simulink model "boostObserver_old"  (R2020a)
settings: Solver=VariableStepAuto  StartTime=0.0  StopTime=3.2  FixedStep=0.0005  MaxStep=9e-06  RelTol=1e-03  EnableMultiTasking=on
InitFcn:
  | kp=0.01;
  | ki=0.01;
  | 
  | k=2;
  | em=100000000;
  | GE=1/em;
  | GU=k*ki/GE;
  | GCE=k*kp/GU;
model workspace (MAT data in the model file):
  time = 0.8
values from neighbouring files (symbols this model uses):
  A1 = obj.boostConverter.A1    [BoostController.m]    (also in BoostConverter.m = [-obj.R/obj.L 0;0 -1/(obj.Ro*obj.C)]; BuckBoostConverter.m = [-obj.R/obj.L 0;0 -1/(obj.Ro*obj.C)]; obsmc.m = Asigma{1,1}; workspace_atual.mat = [-16.4  0; 0  -3.50877192982])
  A2 = obj.boostConverter.A2    [BoostController.m]    (also in BoostConverter.m = [-obj.R/obj.L -1/obj.L;1/obj.C -1/(obj.Ro*obj.C)]; BuckBoostConverter.m = [-obj.R/obj.L 1/obj.L;-1/obj.C -1/(obj.Ro*obj.C)]; obsmc.m = Asigma{1,2}; workspace_atual.mat = [-16.4  -200; 350.877192982  -3.50877192982])
  AlarmDeadTime = 0.50    (= 0.5)    [BoostFaultSimulation.m]    (also in workspace_atual.mat; workspace_certo.mat)
  B1 = obj.boostConverter.B1    [BoostController.m]    (also in BoostConverter.m = [1/obj.L;0]; BuckBoostConverter.m = [1/obj.L;0]; obsmc.m = Bsigma{1,1}; workspace_atual.mat = [200 0])
  boost_parameters = [obj.Ro,obj.R,obj.L,obj.C,obj.u]'    [BoostConverter.m]    (also in BuckBoostConverter.m; boostResults2Latex.m = boost.parameters(); workspace_atual.mat = [100 0.082 0.005 0.00285 190]; workspace_certo.mat = [100 0.082 0.005 0.00285 190])
  C = 1e-3    (= 0.001)    [boostResults2Latex.m]
  CiL = [0 1]    [workspace_atual.mat]    (also in workspace_certo.mat)
  Cmatrix = [1  0; 0  1]    [workspace_atual.mat]    (also in workspace_certo.mat)
  CVc = [1 0]    [workspace_atual.mat]    (also in workspace_certo.mat)
  D1 = [1  0; 0  1]    [workspace_atual.mat]    (also in workspace_certo.mat)
  FaultClass = 0    [BoostFaultSimulation.m]    (also in workspace_atual.mat = 1; workspace_certo.mat = 1)
  iLFaultSwitch = 0    [BoostFaultSimulation.m]    (also in workspace_atual.mat; workspace_certo.mat)
  iLFaultTime = 1.70    (= 1.7)    [BoostFaultSimulation.m]    (also in workspace_atual.mat; workspace_certo.mat)
  iLGainFaultFactor = 15    [BoostFaultSimulation.m]    (also in workspace_atual.mat; workspace_certo.mat)
  iLNoiseFaultSwitch = 0    [BoostFaultSimulation.m]    (also in workspace_atual.mat; workspace_certo.mat)
  iLNoiseTime = 1.70    (= 1.7)    [BoostFaultSimulation.m]    (also in workspace_atual.mat; workspace_certo.mat)
  Jth = 2000    [workspace_atual.mat]    (also in workspace_certo.mat)
  L = 1e-3    (= 0.001)    [boostResults2Latex.m]    (also in obsmc.m = sdpvar(3,1,'full'))
  LoadAddResistor = obj.LoadAddFactor*obj.Ro    [BoostFaultSimulation.m]    (also in workspace_atual.mat = 30; workspace_certo.mat = 30)
  LoadAddSignalSwitch = 1    [BoostFaultSimulation.m]    (also in workspace_atual.mat; workspace_certo.mat)
  LoadAddSwitch = 0    [BoostFaultSimulation.m]    (also in workspace_atual.mat; workspace_certo.mat)
  LoadAddTime = 0.90    (= 0.9)    [BoostFaultSimulation.m]    (also in workspace_atual.mat; workspace_certo.mat)
  LoadRemoveResistor = obj.Ro*(1-obj.LoadRemoveFactor)/(obj.LoadRemoveFactor)    [BoostFaultSimulation.m]    (also in workspace_atual.mat = 233.333333333; workspace_certo.mat = 233.333333333)
  LoadRemoveSignalSwitch = 1    [BoostFaultSimulation.m]    (also in workspace_atual.mat; workspace_certo.mat)
  LoadRemoveSwitch = 0    [BoostFaultSimulation.m]    (also in workspace_atual.mat; workspace_certo.mat)
  LoadRemoveTime = 0.90    (= 0.9)    [BoostFaultSimulation.m]    (also in workspace_atual.mat; workspace_certo.mat)
  LobsiL = [1737913.15707 66180.0912281]    [workspace_atual.mat]    (also in workspace_certo.mat)
  LobsVc = [61200 1]    [workspace_atual.mat]    (also in workspace_certo.mat)
  ObsEp = 70    [workspace_atual.mat]    (also in workspace_certo.mat)
  R = 0.1    [boostResults2Latex.m]    (also in workspace_atual.mat = 0.082; workspace_certo.mat = 0.082)
  ReconfigDelay = 0    [BoostFaultSimulation.m]    (also in workspace_atual.mat = 0.2; workspace_certo.mat = 0.2)
  ReconfigSwitch = 0    [BoostFaultSimulation.m]    (also in workspace_atual.mat; workspace_certo.mat)
  ReconfigTime = 1.707    [BoostFaultSimulation.m]    (also in workspace_atual.mat; workspace_certo.mat)
  rho = 5    [workspace_atual.mat]    (also in workspace_certo.mat)
  RMSfrequency = 47.61    [BoostFaultSimulation.m]    (also in workspace_atual.mat; workspace_certo.mat)
  Ro = 100    [BoostFaultSimulation.m]    (also in boostResults2Latex.m = 10; workspace_atual.mat; workspace_certo.mat)
  Smep = 80    [workspace_atual.mat]    (also in workspace_certo.mat)
  SourceAddSignalSwitch = 1    [BoostFaultSimulation.m]    (also in workspace_atual.mat; workspace_certo.mat)
  SourceAddSwitch = 0    [BoostFaultSimulation.m]    (also in workspace_atual.mat; workspace_certo.mat)
  SourceAddTime = 0.90    (= 0.9)    [BoostFaultSimulation.m]    (also in workspace_atual.mat; workspace_certo.mat)
  SourceAddVoltage = obj.SourceAddFactor*obj.u    [BoostFaultSimulation.m]    (also in workspace_atual.mat = 19; workspace_certo.mat = 19)
  SourceRemoveSignalSwitch = 1    [BoostFaultSimulation.m]    (also in workspace_atual.mat; workspace_certo.mat)
  SourceRemoveSwitch = 0    [BoostFaultSimulation.m]    (also in workspace_atual.mat; workspace_certo.mat)
  SourceRemoveTime = 0.90    (= 0.9)    [BoostFaultSimulation.m]    (also in workspace_atual.mat; workspace_certo.mat)
  SourceRemoveVoltage = obj.SourceRemoveFactor*obj.u    [BoostFaultSimulation.m]    (also in workspace_atual.mat = 19; workspace_certo.mat = 19)
  ueq = 0.5    [workspace_atual.mat]    (also in workspace_certo.mat)
  VcFaultSwitch = 0    [BoostFaultSimulation.m]    (also in workspace_atual.mat; workspace_certo.mat)
  VcFaultTime = 1.70    (= 1.7)    [BoostFaultSimulation.m]    (also in workspace_atual.mat; workspace_certo.mat)
  VcGainFaultFactor = 15    [BoostFaultSimulation.m]    (also in workspace_atual.mat; workspace_certo.mat)
  VcNoiseFaultSwitch = 0    [BoostFaultSimulation.m]    (also in workspace_atual.mat; workspace_certo.mat)
  VcNoiseTime = 1.70    (= 1.7)    [BoostFaultSimulation.m]    (also in workspace_atual.mat; workspace_certo.mat)
  ve = 380    [BoostFaultSimulation.m]    (also in boostResults2Latex.m = 100; workspace_atual.mat; workspace_certo.mat)
  x_e = [ie;ve]    [BoostConverter.m]    (also in BuckBoostConverter.m)
  xe = obj.boostConverter.equilibriumstate(ve)    [BoostController.m]    (also in workspace_atual.mat = [7.62509288104 380]; workspace_certo.mat = [7.62509288104 380])
undefined symbols (not defined in the file or in its folder): Atilde1, Atilde2, Ctilde1, Dtilde1, Dtilde2, F, G, MAXnet, MINnet
libraries: neural x74, powerlib x70, dspstat3 x16, simulink x9, powerlib_meascontrol x7, dspmtrx3 x7, dspmathops x3
(part 3 of 7)

== system boostObserver_old/Subsystem/D(f_s)/Subsystem2 ==
  input : Inport
  FaultStep : Inport  Port=2
  NoiseStep : Inport  Port=3
  FaultSwtich : Inport  Port=4
  NoiseFaultSwitch : Inport  Port=5
  FaultFactor : Inport  Port=6
  Constant11 : Constant  Value=0
  Constant9 : Constant  Value=0
  Product : Product
  Subsystem : Subsystem
  Switch10 : Switch  Criteria=u2 ~= 0
  Switch11 : Switch  Criteria=u2 ~= 0
  Switch13 : Switch  Criteria=u2 ~= 0
  Switch9 : Switch  Criteria=u2 ~= 0  ZeroCross=off
  iLFault Switch : MultiPortSwitch  DataPortOrder=Zero-based contiguous  DataPortForDefault=Additional data port  zeroidx=on
  output : Outport
  wires:
  input/1 -> Product/1, Switch11/3, iLFault Switch/2, Switch10/3, iLFault Switch/5
  Constant9/1 -> Switch10/1
  Switch13/1 -> Switch9/2
  Switch9/1 -> output/1
  Switch11/1 -> iLFault Switch/4
  Constant11/1 -> Switch13/3
  iLFault Switch/1 -> Switch9/3, Subsystem/1(input)
  Switch10/1 -> iLFault Switch/3
  FaultStep/1 -> Switch11/2, Switch10/2
  NoiseStep/1 -> Switch13/1
  FaultSwtich/1 -> iLFault Switch/1
  NoiseFaultSwitch/1 -> Switch13/2
  FaultFactor/1 -> Product/2
  Product/1 -> Switch11/1
  Subsystem/1(noiseOutput) -> Switch9/1

== system boostObserver_old/Subsystem/ErrorGenerator/If Action Subsystem ==
  e_y : Inport
  Action Port : ActionPort  ActionPortLabel=if(u1 ~= 0)
  Matrix Multiply : Product  Multiplication=Matrix(*)
  Matrix Multiply1 : Product
  Matrizes A1 : Constant  Value=rho
  Matrizes A2 : Constant  Value=F
  Normalization : dspmathops/Normalization  NormType=2-norm  Bias=1e-10  NormOver=Each column  Dimension=1  roundingMode=Floor  overflowMode=off  accumDataTypeStr=Inherit: Same as product output  accumLastDataTypeStr=Inherit: Same as product output  outputDataTypeStr=Inherit: Same as product output  outputMin=[]  outputMax=[]  outputLastDataTypeStr=Inherit: Same as product output
  v : Outport
  wires:
  Matrix Multiply/1 -> Normalization/1
  Matrizes A2/1 -> Matrix Multiply/1
  Normalization/1 -> Matrix Multiply1/2
  e_y/1 -> Matrix Multiply/2
  Matrizes A1/1 -> Matrix Multiply1/1
  Matrix Multiply1/1 -> v/1

== system boostObserver_old/Subsystem/ErrorGenerator/If Action Subsystem1 ==
  e_y : Inport
  Action Port : ActionPort  ActionPortLabel=else
  v : Outport
  wires:
  e_y/1 -> v/1

== system boostObserver_old/Subsystem/Fault Identification Neural Netowrk/Pattern Recognition Neural Network1 ==
  Input : Inport  PortDimensions=3
      mask Display: e = 0.06;c1 = [120 230 180]/255;c2 = ([120 230 180]+0)/(256+128);c3 = ([120 230 180]+128)/(256+128);patch([0 1 1 0],[0 0 1 1],c1);patch([0 1 1 1-e 1-e 0+e],[0 0 1 1-e 0+e 0+e],c2);patch([0 0 1 1-e 0+e 0+e],[0 1 1 1-e 1-e 0+e],c3);plot([0 1 1 0 0],[0 0 1 1 0]);
  Layer 1 : Subsystem
      mask Display: e = 0.06;c1 = [120 150 230]/255;c2 = ([120 150 230]+0)/383;c3 = ([120 150 230]+128)/383;patch([0 1 1 0],[0 0 1 1],c1);patch([0 1 1 1-e 1-e 0+e],[0 0 1 1-e 0+e 0+e],c2);patch([0 0 1 1-e 0+e 0+e],[0 1 1 1-e 1-e 0+e],c3);plot([0 1 1 0 0],[0 0 1 1 0]);
  Layer 2 : Subsystem
      mask Display: e = 0.06;c1 = [120 150 230]/255;c2 = ([120 150 230]+0)/383;c3 = ([120 150 230]+128)/383;patch([0 1 1 0],[0 0 1 1],c1);patch([0 1 1 1-e 1-e 0+e],[0 0 1 1-e 0+e 0+e],c2);patch([0 0 1 1-e 0+e 0+e],[0 1 1 1-e 1-e 0+e],c3);plot([0 1 1 0 0],[0 0 1 1 0]);
  Process Input 1 : Subsystem
      mask Display: e = 0.06;c1 = [120 150 230]/255;c2 = ([120 150 230]+0)/383;c3 = ([120 150 230]+128)/383;patch([0 1 1 0],[0 0 1 1],c1);patch([0 1 1 1-e 1-e 0+e],[0 0 1 1-e 0+e 0+e],c2);patch([0 0 1 1-e 0+e 0+e],[0 1 1 1-e 1-e 0+e],c3);plot([0 1 1 0 0],[0 0 1 1 0]);
  Process Output 1 : Subsystem
      mask Display: e = 0.06;c1 = [120 150 230]/255;c2 = ([120 150 230]+0)/383;c3 = ([120 150 230]+128)/383;patch([0 1 1 0],[0 0 1 1],c1);patch([0 1 1 1-e 1-e 0+e],[0 0 1 1-e 0+e 0+e],c2);patch([0 0 1 1-e 0+e 0+e],[0 1 1 1-e 1-e 0+e],c3);plot([0 1 1 0 0],[0 0 1 1 0]);
  Output : Outport  InitialOutput=[0;0;0;0;0]
      mask Display: e = 0.06;c1 = [120 230 180]/255;c2 = ([120 230 180]+0)/(256+128);c3 = ([120 230 180]+128)/(256+128);patch([0 1 1 0],[0 0 1 1],c1);patch([0 1 1 1-e 1-e 0+e],[0 0 1 1-e 0+e 0+e],c2);patch([0 0 1 1-e 0+e 0+e],[0 1 1 1-e 1-e 0+e],c3);plot([0 1 1 0 0],[0 0 1 1 0]);
  wires:
  Input/1 -> Process Input 1/1(x)
  Process Output 1/1(y) -> Output/1
  Process Input 1/1(p) -> Layer 1/1("p{1}")
  Layer 1/1("a{1}") -> [feedback1]
  [feedback1] -> Layer 2/1("a{1} ")
  Layer 2/1("a{2}") -> Process Output 1/1(a)

== system boostObserver_old/Subsystem/Fault Identification Neural Netowrk/Subsystem ==
  input : Inport
  min : Inport  Port=2
  max : Inport  Port=3
  Constant2 : Constant  Value=2
  Constant3 : Constant
  Divide : Product  Inputs=*/
  Product : Product
  Sum : Sum  Inputs=|+-
  Sum1 : Sum  Inputs=|+-
  Sum2 : Sum  Inputs=|+-
  Out1 : Outport
  wires:
  Divide/1 -> Product/2
  max/1 -> Sum2/1
  Constant3/1 -> Sum1/2
  Product/1 -> Sum1/1
  input/1 -> Sum/1
  Sum/1 -> Divide/1
  Sum2/1 -> Divide/2
  Constant2/1 -> Product/1
  Sum1/1 -> Out1/1
  min/1 -> Sum/2, Sum2/2

== system boostObserver_old/Subsystem/Fault Identification Neural Netowrk/Subsystem1 ==
  input : Inport
  min : Inport  Port=2
  max : Inport  Port=3
  Constant2 : Constant  Value=2
  Constant3 : Constant
  Divide : Product  Inputs=*/
  Product : Product
  Sum : Sum  Inputs=|+-
  Sum1 : Sum  Inputs=|+-
  Sum2 : Sum  Inputs=|+-
  Out1 : Outport
  wires:
  Divide/1 -> Product/2
  max/1 -> Sum2/1
  Constant3/1 -> Sum1/2
  Product/1 -> Sum1/1
  input/1 -> Sum/1
  Sum/1 -> Divide/1
  Sum2/1 -> Divide/2
  Constant2/1 -> Product/1
  Sum1/1 -> Out1/1
  min/1 -> Sum/2, Sum2/2

== system boostObserver_old/Subsystem/Fault Identification Neural Netowrk/Subsystem2 ==
  input : Inport
  min : Inport  Port=2
  max : Inport  Port=3
  Constant2 : Constant  Value=2
  Constant3 : Constant
  Divide : Product  Inputs=*/
  Product : Product
  Sum : Sum  Inputs=|+-
  Sum1 : Sum  Inputs=|+-
  Sum2 : Sum  Inputs=|+-
  Out1 : Outport
  wires:
  Divide/1 -> Product/2
  max/1 -> Sum2/1
  Constant3/1 -> Sum1/2
  Product/1 -> Sum1/1
  input/1 -> Sum/1
  Sum/1 -> Divide/1
  Sum2/1 -> Divide/2
  Constant2/1 -> Product/1
  Sum1/1 -> Out1/1
  min/1 -> Sum/2, Sum2/2

== system boostObserver_old/Subsystem/Sliding Mode Observer 5/ObserverDynamics ==
  ey : Inport
  v : Inport  Port=2
  sigma : Inport  Port=3
  Gain : Gain  Gain=Atilde1  Multiplication=Matrix(K*u)
  Gain1 : Gain  Gain=G  Multiplication=Matrix(K*u)
  Gain3 : Gain  Gain=Dtilde1  Multiplication=Matrix(K*u)
  Gain5 : Gain  Gain=Atilde2  Multiplication=Matrix(K*u)
  Gain7 : Gain  Gain=Dtilde2  Multiplication=Matrix(K*u)
  Integral : Subsystem
  Sum : Sum  Inputs=|+++
  Sum1 : Sum  Inputs=|+++
  Switch1 : Switch  Criteria=u2 > Threshold
  e_tilde_hat : Outport
  wires:
  sigma/1 -> Switch1/2
  Switch1/1 -> Integral/1(e_hat_dot)  "v"
  Integral/1(e_hat) -> Gain/1, e_tilde_hat/1, Gain5/1
  ey/1 -> Gain1/1
  v/1 -> Gain7/1, Gain3/1
  Sum1/1 -> Switch1/3
  Sum/1 -> Switch1/1
  Gain7/1 -> Sum1/2
  Gain5/1 -> Sum1/3
  Gain3/1 -> Sum/1
  Gain1/1 -> Sum1/1, Sum/2
  Gain/1 -> Sum/3

== system boostObserver_old/Subsystem/Subsystem/SlidingSurface ==
  S : Inport
  ep : Inport  Port=2
  Abs : Abs  ZeroCross=off
  GreaterThan : RelationalOperator  Operator=>  OutDataTypeStr=boolean  RndMeth=Simplest
  If : If  IfExpression=u1 ~= 0
  If Action Subsystem : Subsystem  TreatAsAtomicUnit=on
  If Action Subsystem2 : Subsystem  TreatAsAtomicUnit=on
  Merge1 : Merge
  d : Outport
  wires:
  If Action Subsystem2/1(d) -> Merge1/2
  [S] -> If Action Subsystem/1(S), If Action Subsystem2/1(S)
  If/2 -> If Action Subsystem2/Action
  If/1 -> If Action Subsystem/Action
  [ep] -> If Action Subsystem2/2(ep)
  S/1 -> [S], Abs/1
  If Action Subsystem/1(d) -> Merge1/1
  Abs/1 -> GreaterThan/1
  GreaterThan/1 -> If/1
  Merge1/1 -> d/1
  ep/1 -> [ep], GreaterThan/2

== system boostObserver_old/Subsystem/Subsystem1/SlidingSurface ==
  S : Inport
  ep : Inport  Port=2
  Abs : Abs  ZeroCross=off
  GreaterThan : RelationalOperator  Operator=>  OutDataTypeStr=boolean  RndMeth=Simplest
  If : If  IfExpression=u1 ~= 0
  If Action Subsystem : Subsystem  TreatAsAtomicUnit=on
  If Action Subsystem2 : Subsystem  TreatAsAtomicUnit=on
  Merge1 : Merge
  d : Outport
  wires:
  If Action Subsystem2/1(d) -> Merge1/2
  [S] -> If Action Subsystem/1(S), If Action Subsystem2/1(S)
  If/2 -> If Action Subsystem2/Action
  If/1 -> If Action Subsystem/Action
  [ep] -> If Action Subsystem2/2(ep)
  S/1 -> [S], Abs/1
  If Action Subsystem/1(d) -> Merge1/1
  Abs/1 -> GreaterThan/1
  GreaterThan/1 -> If/1
  Merge1/1 -> d/1
  ep/1 -> [ep], GreaterThan/2

== system boostObserver_old/Subsystem/Subsystem9/Residual Generator2 ==
  e_y : Inport
  Matrix Square1 : dspmtrx3/Matrix Square  OutMin=[]  OutMax=[]
      settings: SourceProductBaseCode=DS
  Moving RMS : dspstat3/Moving RMS  Method=Sliding window  ForgettingFactorPort=off  SpecifyWindowLength=on  WindowLength=RMSfrequency/10  ForgettingFactor=0.9  SimulateUsing=Code generation
      settings: SourceProductBaseCode=DS
  Sqrt2 : Sqrt  SaturateOnIntegerOverflow=on
  RMS : Outport
  wires:
  Matrix Square1/1 -> Sqrt2/1
  e_y/1 -> Matrix Square1/1
  Sqrt2/1 -> Moving RMS/1
  Moving RMS/1 -> RMS/1

== system boostObserver_old/Subsystem/Vc OBserver/calc_x_hat ==
  sigma : Inport
  rsign : Inport  Port=2
  Lobs : Inport  Port=3
  Gain : Gain  Gain=A1  Multiplication=Matrix(K*u)
  Gain5 : Gain  Gain=A2  Multiplication=Matrix(K*u)
  Integral : Subsystem
  Matrix Multiply : Product  Multiplication=Matrix(*)
  MatrizesA8 : Constant  Value=B1*u
  Scope1 : Scope
  Sum : Sum  Inputs=|+++
  Sum1 : Sum  Inputs=|+++
  Switch1 : Switch  Criteria=u2 ~= 0
  x_hat : Outport
  wires:
  sigma/1 -> Switch1/2
  Switch1/1 -> Integral/1(x_hat_dot)  "v"
  Integral/1(x_hat) -> Scope1/1, x_hat/1, Gain/1, Gain5/1
  Sum1/1 -> Switch1/3
  Sum/1 -> Switch1/1
  Gain/1 -> Sum/3
  Gain5/1 -> Sum1/3
  Matrix Multiply/1 -> Sum/2, Sum1/2
  MatrizesA8/1 -> Sum1/1, Sum/1
  Lobs/1 -> Matrix Multiply/1
  rsign/1 -> Matrix Multiply/2

== system boostObserver_old/Subsystem/iL Observer/calc_x_hat ==
  sigma : Inport
  rsign : Inport  Port=2
  Lobs : Inport  Port=3
  Gain : Gain  Gain=A1  Multiplication=Matrix(K*u)
  Gain5 : Gain  Gain=A2  Multiplication=Matrix(K*u)
  Integral : Subsystem
  Matrix Multiply : Product  Multiplication=Matrix(*)
  MatrizesA8 : Constant  Value=B1*u
  Scope1 : Scope
  Sum : Sum  Inputs=|+++
  Sum1 : Sum  Inputs=|+++
  Switch1 : Switch  Criteria=u2 ~= 0
  x_hat : Outport
  wires:
  sigma/1 -> Switch1/2
  Switch1/1 -> Integral/1(x_hat_dot)  "v"
  Integral/1(x_hat) -> Scope1/1, x_hat/1, Gain/1, Gain5/1
  Sum1/1 -> Switch1/3
  Sum/1 -> Switch1/1
  Gain/1 -> Sum/3
  Gain5/1 -> Sum1/3
  Matrix Multiply/1 -> Sum/2, Sum1/2
  MatrizesA8/1 -> Sum1/1, Sum/1
  Lobs/1 -> Matrix Multiply/1
  rsign/1 -> Matrix Multiply/2

== system boostObserver_old/Subsystem3/Augmented Error Generator/z1 ==
  z_dot : Inport
  Constant1 : Constant  Value=[0;0]  VectorParams1D=off
  Gain2 : Gain  Gain=Cmatrix  Multiplication=Matrix(K*u) (u vector)
  Integrator6 : Integrator  InitialConditionSource=external
  z : Outport
  wires:
  Gain2/1 -> Integrator6/1
  Integrator6/1 -> z/1
  z_dot/1 -> Gain2/1
  Constant1/1 -> Integrator6/2

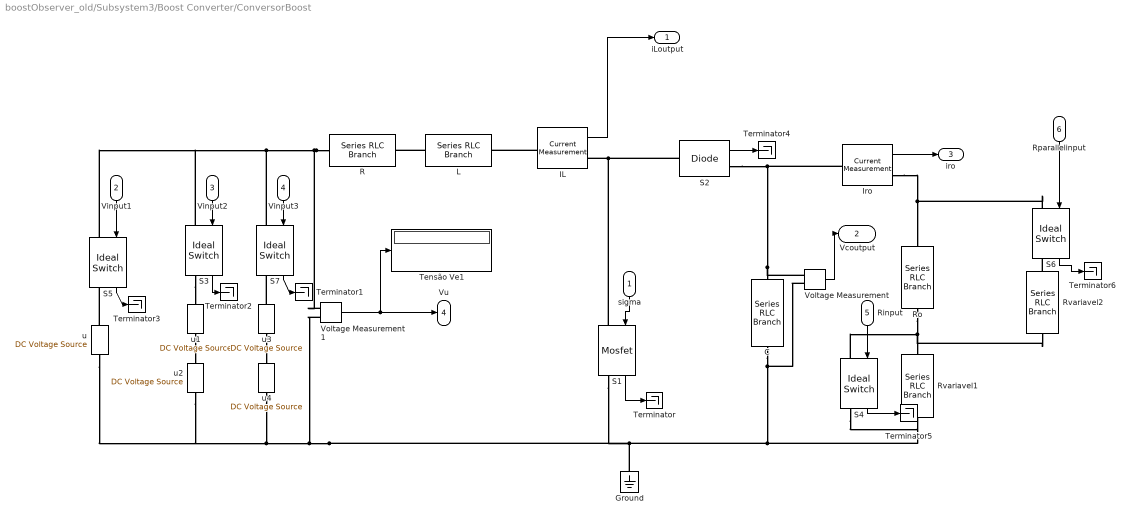
== system boostObserver_old/Subsystem3/Boost Converter/ConversorBoost ==
  sigma : Inport
  Vinput1 : Inport  Port=2
  Vinput2 : Inport  Port=3
  Vinput3 : Inport  Port=4
  Rinput : Inport  Port=5
  Rparallelinput : Inport  Port=6
  C : powerlib/Elements/Series RLC Branch  LConnTagsString=__new0  RConnTagsString=__new0  BranchType=C  Resistance=1  Inductance=1e-3  SetiL0=off  InitialCurrent=0  Capacitance=C  Setx0=on  InitialVoltage=0  Measurements=None
  Ground : powerlib/Elements/Ground  LConnTagsString=a
  IL : powerlib/Measurements/Current Measurement  PhasorSimulation=off  OutputType=Complex  PSBequivalent=0
  Iro : powerlib/Measurements/Current Measurement  PhasorSimulation=off  OutputType=Complex  PSBequivalent=0
  L : powerlib/Elements/Series RLC Branch  LConnTagsString=__new0  RConnTagsString=__new0  BranchType=L  Resistance=1  Inductance=L  SetiL0=on  InitialCurrent=0  Capacitance=1e-6  Setx0=off  InitialVoltage=0  Measurements=None
  R : powerlib/Elements/Series RLC Branch  LConnTagsString=__new0  RConnTagsString=__new0  BranchType=R  Resistance=R  Inductance=1e-3  SetiL0=off  InitialCurrent=0  Capacitance=1e-6  Setx0=off  InitialVoltage=0  Measurements=None
  Ro : powerlib/Elements/Series RLC Branch  LConnTagsString=__new0  RConnTagsString=__new0  BranchType=R  Resistance=Ro  Inductance=1e-3  SetiL0=off  InitialCurrent=0  Capacitance=1e-6  Setx0=off  InitialVoltage=0  Measurements=None
  Rvariavel1 : powerlib/Elements/Series RLC Branch  LConnTagsString=__new0  RConnTagsString=__new0  BranchType=R  Resistance=LoadAddResistor  Inductance=1e-3  SetiL0=off  InitialCurrent=0  Capacitance=1e-6  Setx0=off  InitialVoltage=0  Measurements=None
  Rvariavel2 : powerlib/Elements/Series RLC Branch  LConnTagsString=__new0  RConnTagsString=__new0  BranchType=R  Resistance=LoadRemoveResistor  Inductance=1e-3  SetiL0=off  InitialCurrent=0  Capacitance=1e-6  Setx0=off  InitialVoltage=0  Measurements=None
  S1 : powerlib/Power Electronics/Mosfet  Ron=0.0000001  Lon=0  Rd=0.000000001  Vfd=0  IC=0  Rs=1e5  Cs=inf  Measurements=on
  S2 : powerlib/Power Electronics/Diode  Ron=0.000001  Lon=0  Vf=0  IC=0  UseSnubber=off  Rs=0  Cs=0  Measurements=on
  S{3..7} (5 alike) : powerlib/Power Electronics/Ideal Switch  Ron=0.0000001  Lon=0  IC=0  Rs=1e8  Cs=inf  Measurements=on
  Tensão Ve1 : Display
  Terminator{,1..6} (7 alike) : Terminator
  Voltage Measurement : powerlib/Measurements/Voltage Measurement  PhasorSimulation=off  OutputType=Complex  PSBequivalent=0
  Voltage Measurement1 : powerlib/Measurements/Voltage Measurement  PhasorSimulation=off  OutputType=Complex  PSBequivalent=0
  u : powerlib/Electrical Sources/DC Voltage Source  Amplitude=u  Measurements=None
  u1 : powerlib/Electrical Sources/DC Voltage Source  Amplitude=SourceAddVoltage  Measurements=None
  u2 : powerlib/Electrical Sources/DC Voltage Source  Amplitude=u  Measurements=None
  u3 : powerlib/Electrical Sources/DC Voltage Source  Amplitude=SourceRemoveVoltage  Measurements=None
  u4 : powerlib/Electrical Sources/DC Voltage Source  Amplitude=u  Measurements=None
  iLoutput : Outport
  Vcoutput : Outport  Port=2
  iro : Outport  Port=3
  Vu : Outport  Port=4
  wires:
  Rinput/1 -> S4/1
  IL/1 -> iLoutput/1
  sigma/1 -> S1/1
  Voltage Measurement/1 -> Vcoutput/1
  Iro/1 -> iro/1
  Voltage Measurement1/1 -> Vu/1, Tensão Ve1/1
  Vinput1/1 -> S5/1
  Vinput2/1 -> S3/1
  Rparallelinput/1 -> S6/1
  Vinput3/1 -> S7/1
  S1/1 -> Terminator/1
  S7/1 -> Terminator1/1
  S3/1 -> Terminator2/1
  S5/1 -> Terminator3/1
  S2/1 -> Terminator4/1
  S4/1 -> Terminator5/1
  S6/1 -> Terminator6/1
  connections:
  Ro/RConn1 -- Rvariavel2/LConn1 -- Rvariavel1/RConn1 -- S4/LConn1
  IL/LConn1 -- L/RConn1
  C/RConn1 -- S4/RConn1 -- Rvariavel1/LConn1 -- S1/RConn1 -- u2/LConn1 -- u/LConn1 -- u4/LConn1 -- Voltage Measurement1/LConn2 -- Ground/LConn1 -- Voltage Measurement/LConn2
  S2/LConn1 -- S1/LConn1 -- IL/RConn1
  R/LConn1 -- S3/LConn1 -- S5/LConn1 -- S7/LConn1 -- Voltage Measurement1/LConn1
  Iro/RConn1 -- S6/LConn1 -- Ro/LConn1
  L/LConn1 -- R/RConn1
  S2/RConn1 -- Iro/LConn1 -- Voltage Measurement/LConn1 -- C/LConn1
  u/RConn1 -- S5/RConn1
  Rvariavel2/RConn1 -- S6/RConn1
  S3/RConn1 -- u1/RConn1
  u1/LConn1 -- u2/RConn1
  u3/LConn1 -- S7/RConn1
  u3/RConn1 -- u4/RConn1

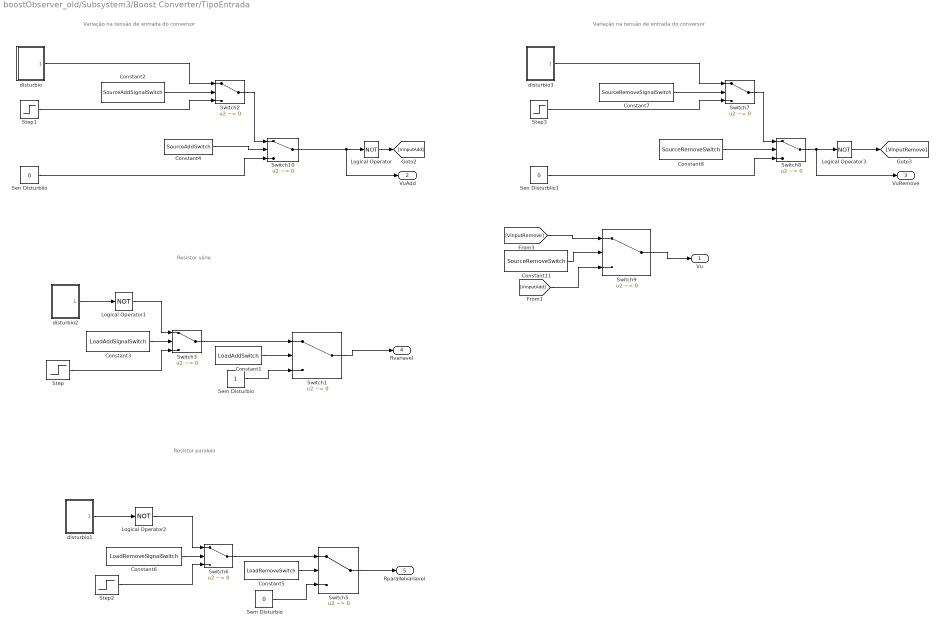
== system boostObserver_old/Subsystem3/Boost Converter/TipoEntrada ==
  note: Variação na tensão de entrada do conversor
  note: Resistor série
  note: Resistor paralelo
  note: Variação na tensão de entrada do conversor
  Constant1 : Constant  Value=LoadAddSwitch
  Constant11 : Constant  Value=SourceRemoveSwitch
  Constant2 : Constant  Value=SourceAddSignalSwitch
  Constant3 : Constant  Value=LoadAddSignalSwitch
  Constant4 : Constant  Value=SourceAddSwitch
  Constant5 : Constant  Value=LoadRemoveSwitch
  Constant6 : Constant  Value=LoadRemoveSignalSwitch
  Constant7 : Constant  Value=SourceRemoveSignalSwitch
  Constant8 : Constant  Value=SourceRemoveSwitch
  Logical Operator{,1..3} (4 alike) : Logic  Operator=NOT  AllPortsSameDT=off  OutDataTypeStr=boolean
  Sem Disturbio : Constant
  "Sem Disturbio  " : Constant  Value=0
  Sen Disturbiio : Constant  Value=0
  Sen Disturbiio1 : Constant  Value=0
  Step : Step  Time=LoadAddTime  Before=1  After=0  SampleTime=0
  Step1 : Step  Time=SourceAddTime  SampleTime=0
  Step2 : Step  Time=LoadRemoveTime  SampleTime=0
  Step3 : Step  Time=SourceRemoveTime  SampleTime=0
  Switch{1..3,5..10} (9 alike) : Switch  Criteria=u2 ~= 0
  disturbio : Subsystem
  disturbio1 : Subsystem
  disturbio2 : Subsystem
  disturbio3 : Subsystem
  Vu : Outport
  VuAdd : Outport  Port=2
  VuRemove : Outport  Port=3
  "Rvariavel " : Outport  Port=4
  "Rparallelvariavel " : Outport  Port=5
  wires:
  Sen Disturbiio/1 -> Switch10/3
  Constant4/1 -> Switch10/2
  Constant1/1 -> Switch1/2
  Switch1/1 -> "Rvariavel "/1
  Constant2/1 -> Switch2/2
  Constant3/1 -> Switch3/2
  Switch2/1 -> Switch10/1
  disturbio2/1(disturbio) -> Logical Operator1/1
  Switch3/1 -> Switch1/1
  Sem Disturbio/1 -> Switch1/3
  Switch6/1 -> Switch5/1
  disturbio1/1(disturbio) -> Logical Operator2/1
  Constant6/1 -> Switch6/2
  "Sem Disturbio  "/1 -> Switch5/3
  Switch5/1 -> "Rparallelvariavel "/1
  Constant5/1 -> Switch5/2
  disturbio/1(disturbio) -> Switch2/1
  Step1/1 -> Switch2/3
  Logical Operator1/1 -> Switch3/1
  Step/1 -> Switch3/3
  Step2/1 -> Switch6/3
  Logical Operator2/1 -> Switch6/1
  disturbio3/1(disturbio) -> Switch7/1
  Constant8/1 -> Switch8/2
  Constant7/1 -> Switch7/2
  Switch8/1 -> VuRemove/1, Logical Operator3/1
  Sen Disturbiio1/1 -> Switch8/3
  Switch7/1 -> Switch8/1
  Step3/1 -> Switch7/3
  [VinputAdd] -> Switch9/3
  Constant11/1 -> Switch9/2
  Switch10/1 -> VuAdd/1, Logical Operator/1
  Switch9/1 -> Vu/1
  Logical Operator/1 -> [VinputAdd]
  Logical Operator3/1 -> [VinputRemove]
  [VinputRemove] -> Switch9/1

== system boostObserver_old/Subsystem3/Controlador1/SlidingSurface ==
  S : Inport
  ep : Inport  Port=2
  Abs : Abs
  GreaterThan : RelationalOperator  Operator=>  OutDataTypeStr=boolean  RndMeth=Simplest
  If : If  IfExpression=u1 ~= 0
  If Action Subsystem : Subsystem  TreatAsAtomicUnit=on
  If Action Subsystem2 : Subsystem  TreatAsAtomicUnit=on
  Merge1 : Merge
  d : Outport
  wires:
  If Action Subsystem2/1(d) -> Merge1/2
  [S] -> If Action Subsystem/1(S), If Action Subsystem2/1(S)
  If/2 -> If Action Subsystem2/Action
  If/1 -> If Action Subsystem/Action
  [ep] -> If Action Subsystem2/2(ep)
  S/1 -> [S], Abs/1
  If Action Subsystem/1(d) -> Merge1/1
  Abs/1 -> GreaterThan/1
  GreaterThan/1 -> If/1
  Merge1/1 -> d/1
  ep/1 -> [ep], GreaterThan/2

== system boostObserver_old/Subsystem3/D(f_s)/Subsystem ==
  input : Inport
  FaultStep : Inport  Port=2
  NoiseStep : Inport  Port=3
  FaultSwtich : Inport  Port=4
  NoiseFaultSwitch : Inport  Port=5
  FaultFactor : Inport  Port=6
  Constant11 : Constant  Value=0
  Constant9 : Constant  Value=0
  Product : Product
  Subsystem : Subsystem
  Switch{9..11,13} (4 alike) : Switch  Criteria=u2 ~= 0
  iLFault Switch : MultiPortSwitch  DataPortOrder=Zero-based contiguous  DataPortForDefault=Additional data port  zeroidx=on
  output : Outport
  wires:
  input/1 -> Product/1, Switch11/3, Switch10/3, iLFault Switch/2, iLFault Switch/5
  Constant9/1 -> Switch10/1
  Switch13/1 -> Switch9/2
  Switch9/1 -> output/1
  Switch11/1 -> iLFault Switch/4
  Constant11/1 -> Switch13/3
  iLFault Switch/1 -> Switch9/3, Subsystem/1(input)
  Switch10/1 -> iLFault Switch/3
  FaultStep/1 -> Switch10/2, Switch11/2
  NoiseStep/1 -> Switch13/1
  FaultSwtich/1 -> iLFault Switch/1
  NoiseFaultSwitch/1 -> Switch13/2
  Product/1 -> Switch11/1
  FaultFactor/1 -> Product/2
  Subsystem/1(noiseOutput) -> Switch9/1

== system boostObserver_old/Subsystem3/D(f_s)/Subsystem2 ==
  input : Inport
  FaultStep : Inport  Port=2
  NoiseStep : Inport  Port=3
  FaultSwtich : Inport  Port=4
  NoiseFaultSwitch : Inport  Port=5
  FaultFactor : Inport  Port=6
  Constant11 : Constant  Value=0
  Constant9 : Constant  Value=0
  Product : Product
  Subsystem : Subsystem
  Switch10 : Switch  Criteria=u2 ~= 0
  Switch11 : Switch  Criteria=u2 ~= 0
  Switch13 : Switch  Criteria=u2 ~= 0
  Switch9 : Switch  Criteria=u2 ~= 0  ZeroCross=off
  iLFault Switch : MultiPortSwitch  DataPortOrder=Zero-based contiguous  DataPortForDefault=Additional data port  zeroidx=on
  output : Outport
  wires:
  input/1 -> Product/1, Switch11/3, iLFault Switch/2, Switch10/3, iLFault Switch/5
  Constant9/1 -> Switch10/1
  Switch13/1 -> Switch9/2
  Switch9/1 -> output/1
  Switch11/1 -> iLFault Switch/4
  Constant11/1 -> Switch13/3
  iLFault Switch/1 -> Switch9/3, Subsystem/1(input)
  Switch10/1 -> iLFault Switch/3
  FaultStep/1 -> Switch11/2, Switch10/2
  NoiseStep/1 -> Switch13/1
  FaultSwtich/1 -> iLFault Switch/1
  NoiseFaultSwitch/1 -> Switch13/2
  FaultFactor/1 -> Product/2
  Product/1 -> Switch11/1
  Subsystem/1(noiseOutput) -> Switch9/1

== system boostObserver_old/Subsystem3/ErrorGenerator/If Action Subsystem ==
  e_y : Inport
  Action Port : ActionPort
  Matrix Multiply : Product  Multiplication=Matrix(*)
  Matrix Multiply1 : Product
  Matrizes A1 : Constant  Value=rho
  Matrizes A2 : Constant  Value=F
  Normalization : dspmathops/Normalization  NormType=2-norm  Bias=1e-10  NormOver=Each column  Dimension=1  roundingMode=Floor  overflowMode=off  accumDataTypeStr=Inherit: Same as product output  accumLastDataTypeStr=Inherit: Same as product output  outputDataTypeStr=Inherit: Same as product output  outputMin=[]  outputMax=[]  outputLastDataTypeStr=Inherit: Same as product output
  v : Outport
  wires:
  Matrix Multiply/1 -> Normalization/1
  Matrizes A2/1 -> Matrix Multiply/1
  Normalization/1 -> Matrix Multiply1/2
  e_y/1 -> Matrix Multiply/2
  Matrizes A1/1 -> Matrix Multiply1/1
  Matrix Multiply1/1 -> v/1

== system boostObserver_old/Subsystem3/ErrorGenerator/If Action Subsystem1 ==
  e_y : Inport
  Action Port : ActionPort
  v : Outport
  wires:
  e_y/1 -> v/1

== system boostObserver_old/Subsystem3/Fault Identification Neural Netowrk/Pattern Recognition Neural Network ==
  Input : Inport  PortDimensions=3
      mask Display: e = 0.06;c1 = [120 230 180]/255;c2 = ([120 230 180]+0)/(256+128);c3 = ([120 230 180]+128)/(256+128);patch([0 1 1 0],[0 0 1 1],c1);patch([0 1 1 1-e 1-e 0+e],[0 0 1 1-e 0+e 0+e],c2);patch([0 0 1 1-e 0+e 0+e],[0 1 1 1-e 1-e 0+e],c3);plot([0 1 1 0 0],[0 0 1 1 0]);
  Layer 1 : Subsystem
      mask Display: e = 0.06;c1 = [120 150 230]/255;c2 = ([120 150 230]+0)/383;c3 = ([120 150 230]+128)/383;patch([0 1 1 0],[0 0 1 1],c1);patch([0 1 1 1-e 1-e 0+e],[0 0 1 1-e 0+e 0+e],c2);patch([0 0 1 1-e 0+e 0+e],[0 1 1 1-e 1-e 0+e],c3);plot([0 1 1 0 0],[0 0 1 1 0]);
  Layer 2 : Subsystem
      mask Display: e = 0.06;c1 = [120 150 230]/255;c2 = ([120 150 230]+0)/383;c3 = ([120 150 230]+128)/383;patch([0 1 1 0],[0 0 1 1],c1);patch([0 1 1 1-e 1-e 0+e],[0 0 1 1-e 0+e 0+e],c2);patch([0 0 1 1-e 0+e 0+e],[0 1 1 1-e 1-e 0+e],c3);plot([0 1 1 0 0],[0 0 1 1 0]);
  Process Input 1 : Subsystem
      mask Display: e = 0.06;c1 = [120 150 230]/255;c2 = ([120 150 230]+0)/383;c3 = ([120 150 230]+128)/383;patch([0 1 1 0],[0 0 1 1],c1);patch([0 1 1 1-e 1-e 0+e],[0 0 1 1-e 0+e 0+e],c2);patch([0 0 1 1-e 0+e 0+e],[0 1 1 1-e 1-e 0+e],c3);plot([0 1 1 0 0],[0 0 1 1 0]);
  Process Output 1 : Subsystem
      mask Display: e = 0.06;c1 = [120 150 230]/255;c2 = ([120 150 230]+0)/383;c3 = ([120 150 230]+128)/383;patch([0 1 1 0],[0 0 1 1],c1);patch([0 1 1 1-e 1-e 0+e],[0 0 1 1-e 0+e 0+e],c2);patch([0 0 1 1-e 0+e 0+e],[0 1 1 1-e 1-e 0+e],c3);plot([0 1 1 0 0],[0 0 1 1 0]);
  Output : Outport  InitialOutput=[0;0;0;0;0;0]
      mask Display: e = 0.06;c1 = [120 230 180]/255;c2 = ([120 230 180]+0)/(256+128);c3 = ([120 230 180]+128)/(256+128);patch([0 1 1 0],[0 0 1 1],c1);patch([0 1 1 1-e 1-e 0+e],[0 0 1 1-e 0+e 0+e],c2);patch([0 0 1 1-e 0+e 0+e],[0 1 1 1-e 1-e 0+e],c3);plot([0 1 1 0 0],[0 0 1 1 0]);
  wires:
  Input/1 -> Process Input 1/1(x)
  Process Output 1/1(y) -> Output/1
  Process Input 1/1(p) -> Layer 1/1("p{1}")
  Layer 1/1("a{1}") -> [feedback1]
  [feedback1] -> Layer 2/1("a{1} ")
  Layer 2/1("a{2}") -> Process Output 1/1(a)

== system boostObserver_old/Subsystem3/Fault Identification Neural Netowrk/Pattern Recognition Neural Network Reconfig Big Data ==
  Input : Inport  PortDimensions=3
      mask Display: e = 0.06;c1 = [120 230 180]/255;c2 = ([120 230 180]+0)/(256+128);c3 = ([120 230 180]+128)/(256+128);patch([0 1 1 0],[0 0 1 1],c1);patch([0 1 1 1-e 1-e 0+e],[0 0 1 1-e 0+e 0+e],c2);patch([0 0 1 1-e 0+e 0+e],[0 1 1 1-e 1-e 0+e],c3);plot([0 1 1 0 0],[0 0 1 1 0]);
  Layer 1 : Subsystem
      mask Display: e = 0.06;c1 = [120 150 230]/255;c2 = ([120 150 230]+0)/383;c3 = ([120 150 230]+128)/383;patch([0 1 1 0],[0 0 1 1],c1);patch([0 1 1 1-e 1-e 0+e],[0 0 1 1-e 0+e 0+e],c2);patch([0 0 1 1-e 0+e 0+e],[0 1 1 1-e 1-e 0+e],c3);plot([0 1 1 0 0],[0 0 1 1 0]);
  Layer 2 : Subsystem
      mask Display: e = 0.06;c1 = [120 150 230]/255;c2 = ([120 150 230]+0)/383;c3 = ([120 150 230]+128)/383;patch([0 1 1 0],[0 0 1 1],c1);patch([0 1 1 1-e 1-e 0+e],[0 0 1 1-e 0+e 0+e],c2);patch([0 0 1 1-e 0+e 0+e],[0 1 1 1-e 1-e 0+e],c3);plot([0 1 1 0 0],[0 0 1 1 0]);
  Process Input 1 : Subsystem
      mask Display: e = 0.06;c1 = [120 150 230]/255;c2 = ([120 150 230]+0)/383;c3 = ([120 150 230]+128)/383;patch([0 1 1 0],[0 0 1 1],c1);patch([0 1 1 1-e 1-e 0+e],[0 0 1 1-e 0+e 0+e],c2);patch([0 0 1 1-e 0+e 0+e],[0 1 1 1-e 1-e 0+e],c3);plot([0 1 1 0 0],[0 0 1 1 0]);
  Process Output 1 : Subsystem
      mask Display: e = 0.06;c1 = [120 150 230]/255;c2 = ([120 150 230]+0)/383;c3 = ([120 150 230]+128)/383;patch([0 1 1 0],[0 0 1 1],c1);patch([0 1 1 1-e 1-e 0+e],[0 0 1 1-e 0+e 0+e],c2);patch([0 0 1 1-e 0+e 0+e],[0 1 1 1-e 1-e 0+e],c3);plot([0 1 1 0 0],[0 0 1 1 0]);
  Output : Outport  InitialOutput=[0;0;0;0;0;0]
      mask Display: e = 0.06;c1 = [120 230 180]/255;c2 = ([120 230 180]+0)/(256+128);c3 = ([120 230 180]+128)/(256+128);patch([0 1 1 0],[0 0 1 1],c1);patch([0 1 1 1-e 1-e 0+e],[0 0 1 1-e 0+e 0+e],c2);patch([0 0 1 1-e 0+e 0+e],[0 1 1 1-e 1-e 0+e],c3);plot([0 1 1 0 0],[0 0 1 1 0]);
  wires:
  Input/1 -> Process Input 1/1(x)
  Process Output 1/1(y) -> Output/1
  Process Input 1/1(p) -> Layer 1/1("p{1}")
  Layer 1/1("a{1}") -> [feedback1]
  [feedback1] -> Layer 2/1("a{1} ")
  Layer 2/1("a{2}") -> Process Output 1/1(a)

== system boostObserver_old/Subsystem3/If Action Subsystem1/GetInitialTime ==
  Clock : Inport
  Constant2 : Constant  Value=0
  Constant3 : Constant
  Constant4 : Constant  Value=0
  Edge Detector : powerlib_meascontrol/Logic/Edge Detector  model=Rising  ic=0  Ts=0
      settings: SourceProductBaseCode=PS
  If : If
  If Action Subsystem : Subsystem  TreatAsAtomicUnit=on
  If Action Subsystem1 : Subsystem  TreatAsAtomicUnit=on
  Memory : Memory
  Merge : Merge
  Switch : Switch  Criteria=u2 > Threshold
  Switch1 : Switch  Criteria=u2 > Threshold
  InitialTime : Outport
  wires:
  If/2 -> If Action Subsystem1/Action
  Memory/1 -> Switch1/3
  Constant3/1 -> Switch/1
  Switch1/1 -> InitialTime/1, Memory/1
  Merge/1 -> Switch1/2, Switch1/1
  Constant4/1 -> Switch/3
  Switch/1 -> If/1
  Constant2/1 -> If Action Subsystem1/1(In1)
  Clock/1 -> [Clock], Edge Detector/1
  If Action Subsystem/1(Out1) -> Merge/2
  Edge Detector/1 -> Switch/2
  [Clock] -> If Action Subsystem/1(In1)
  If/1 -> If Action Subsystem/Action
  If Action Subsystem1/1(Out1) -> Merge/1

== system boostObserver_old/Subsystem3/If Action Subsystem4/GetInitialTime ==
  Clock : Inport
  Constant2 : Constant  Value=0
  Constant3 : Constant
  Constant4 : Constant  Value=0
  Edge Detector : powerlib_meascontrol/Logic/Edge Detector  model=Rising  ic=0  Ts=0
      settings: SourceProductBaseCode=PS
  If : If
  If Action Subsystem : Subsystem  TreatAsAtomicUnit=on
  If Action Subsystem1 : Subsystem  TreatAsAtomicUnit=on
  Memory : Memory
  Merge : Merge
  Switch : Switch  Criteria=u2 > Threshold
  Switch1 : Switch  Criteria=u2 > Threshold
  InitialTime : Outport
  wires:
  If/2 -> If Action Subsystem1/Action
  Memory/1 -> Switch1/3
  Constant3/1 -> Switch/1
  Switch1/1 -> InitialTime/1, Memory/1
  Merge/1 -> Switch1/2, Switch1/1
  Constant4/1 -> Switch/3
  Switch/1 -> If/1
  Constant2/1 -> If Action Subsystem1/1(In1)
  Clock/1 -> [Clock], Edge Detector/1
  If Action Subsystem/1(Out1) -> Merge/2
  Edge Detector/1 -> Switch/2
  [Clock] -> If Action Subsystem/1(In1)
  If/1 -> If Action Subsystem/Action
  If Action Subsystem1/1(Out1) -> Merge/1

== system boostObserver_old/Subsystem3/Residual Generator/Residual Generator1 ==
  e_y : Inport
  Matrix Square1 : dspmtrx3/Matrix Square  OutMin=[]  OutMax=[]
      settings: SourceProductBaseCode=DS
  Moving RMS : dspstat3/Moving RMS  Method=Sliding window  ForgettingFactorPort=off  SpecifyWindowLength=on  WindowLength=RMSfrequency  ForgettingFactor=0.9  SimulateUsing=Code generation
      settings: SourceProductBaseCode=DS
  Sqrt2 : Sqrt  SaturateOnIntegerOverflow=on
  RMS : Outport
  wires:
  Matrix Square1/1 -> Sqrt2/1
  Sqrt2/1 -> Moving RMS/1
  e_y/1 -> Matrix Square1/1
  Moving RMS/1 -> RMS/1

== system boostObserver_old/Subsystem3/Sliding Mode Observer 5/ObserverDynamics ==
  ey : Inport
  v : Inport  Port=2
  sigma : Inport  Port=3
  Gain : Gain  Gain=Atilde1  Multiplication=Matrix(K*u)
  Gain1 : Gain  Gain=G  Multiplication=Matrix(K*u)
  Gain3 : Gain  Gain=Dtilde1  Multiplication=Matrix(K*u)
  Gain5 : Gain  Gain=Atilde2  Multiplication=Matrix(K*u)
  Gain7 : Gain  Gain=Dtilde2  Multiplication=Matrix(K*u)
  Integral : Subsystem
  Sum : Sum  Inputs=|+++
  Sum1 : Sum  Inputs=|+++
  Switch1 : Switch  Criteria=u2 > Threshold
  e_tilde_hat : Outport
  wires:
  sigma/1 -> Switch1/2
  Switch1/1 -> Integral/1(e_hat_dot)  "v"
  Integral/1(e_hat) -> Gain/1, e_tilde_hat/1, Gain5/1
  ey/1 -> Gain1/1
  v/1 -> Gain7/1, Gain3/1
  Sum1/1 -> Switch1/3
  Sum/1 -> Switch1/1
  Gain7/1 -> Sum1/2
  Gain5/1 -> Sum1/3
  Gain3/1 -> Sum/1
  Gain1/1 -> Sum1/1, Sum/2
  Gain/1 -> Sum/3

== system boostObserver_old/Subsystem3/Subsystem/SlidingSurface ==
  S : Inport
  ep : Inport  Port=2
  Abs : Abs  ZeroCross=off
  GreaterThan : RelationalOperator  Operator=>  OutDataTypeStr=boolean  RndMeth=Simplest
  If : If  IfExpression=u1 ~= 0
  If Action Subsystem : Subsystem  TreatAsAtomicUnit=on
  If Action Subsystem2 : Subsystem  TreatAsAtomicUnit=on
  Merge1 : Merge
  d : Outport
  wires:
  If Action Subsystem2/1(d) -> Merge1/2
  [S] -> If Action Subsystem/1(S), If Action Subsystem2/1(S)
  If/2 -> If Action Subsystem2/Action
  If/1 -> If Action Subsystem/Action
  [ep] -> If Action Subsystem2/2(ep)
  S/1 -> [S], Abs/1
  If Action Subsystem/1(d) -> Merge1/1
  Abs/1 -> GreaterThan/1
  GreaterThan/1 -> If/1
  Merge1/1 -> d/1
  ep/1 -> [ep], GreaterThan/2

== system boostObserver_old/Subsystem3/Subsystem1/SlidingSurface ==
  S : Inport
  ep : Inport  Port=2
  Abs : Abs  ZeroCross=off
  GreaterThan : RelationalOperator  Operator=>  OutDataTypeStr=boolean  RndMeth=Simplest
  If : If  IfExpression=u1 ~= 0
  If Action Subsystem : Subsystem  TreatAsAtomicUnit=on
  If Action Subsystem2 : Subsystem  TreatAsAtomicUnit=on
  Merge1 : Merge
  d : Outport
  wires:
  If Action Subsystem2/1(d) -> Merge1/2
  [S] -> If Action Subsystem/1(S), If Action Subsystem2/1(S)
  If/2 -> If Action Subsystem2/Action
  If/1 -> If Action Subsystem/Action
  [ep] -> If Action Subsystem2/2(ep)
  S/1 -> [S], Abs/1
  If Action Subsystem/1(d) -> Merge1/1
  Abs/1 -> GreaterThan/1
  GreaterThan/1 -> If/1
  Merge1/1 -> d/1
  ep/1 -> [ep], GreaterThan/2

== system boostObserver_old/Subsystem3/Subsystem9/Residual Generator1 ==
  e_y : Inport
  Moving RMS : dspstat3/Moving RMS  Method=Sliding window  ForgettingFactorPort=off  SpecifyWindowLength=on  WindowLength=RMSfrequency  ForgettingFactor=0.9  SimulateUsing=Code generation
      settings: SourceProductBaseCode=DS
  RMS : Outport
  wires:
  e_y/1 -> Moving RMS/1
  Moving RMS/1 -> RMS/1

== system boostObserver_old/Subsystem3/Subsystem9/Residual Generator2 ==
  e_y : Inport
  Moving RMS : dspstat3/Moving RMS  Method=Sliding window  ForgettingFactorPort=off  SpecifyWindowLength=on  WindowLength=RMSfrequency  ForgettingFactor=0.9  SimulateUsing=Code generation
      settings: SourceProductBaseCode=DS
  RMS : Outport
  wires:
  e_y/1 -> Moving RMS/1
  Moving RMS/1 -> RMS/1

== system boostObserver_old/Subsystem3/Vc OBserver/calc_x_hat ==
  sigma : Inport
  rsign : Inport  Port=2
  Lobs : Inport  Port=3
  Gain : Gain  Gain=A1  Multiplication=Matrix(K*u)
  Gain5 : Gain  Gain=A2  Multiplication=Matrix(K*u)
  Integral : Subsystem
  Matrix Multiply : Product  Multiplication=Matrix(*)
  MatrizesA8 : Constant  Value=B1*u
  Scope1 : Scope
  Sum : Sum  Inputs=|+++
  Sum1 : Sum  Inputs=|+++
  Switch1 : Switch  Criteria=u2 ~= 0
  x_hat : Outport
  wires:
  sigma/1 -> Switch1/2
  Switch1/1 -> Integral/1(x_hat_dot)  "v"
  Integral/1(x_hat) -> Scope1/1, x_hat/1, Gain/1, Gain5/1
  Sum1/1 -> Switch1/3
  Sum/1 -> Switch1/1
  Gain/1 -> Sum/3
  Gain5/1 -> Sum1/3
  Matrix Multiply/1 -> Sum/2, Sum1/2
  MatrizesA8/1 -> Sum1/1, Sum/1
  Lobs/1 -> Matrix Multiply/1
  rsign/1 -> Matrix Multiply/2

== system boostObserver_old/Subsystem3/iL Observer/calc_x_hat ==
  sigma : Inport
  rsign : Inport  Port=2
  Lobs : Inport  Port=3
  Gain : Gain  Gain=A1  Multiplication=Matrix(K*u)
  Gain5 : Gain  Gain=A2  Multiplication=Matrix(K*u)
  Integral : Subsystem
  Matrix Multiply : Product  Multiplication=Matrix(*)
  MatrizesA8 : Constant  Value=B1*u
  Scope1 : Scope
  Sum : Sum  Inputs=|+++
  Sum1 : Sum  Inputs=|+++
  Switch1 : Switch  Criteria=u2 ~= 0
  x_hat : Outport
  wires:
  sigma/1 -> Switch1/2
  Switch1/1 -> Integral/1(x_hat_dot)  "v"
  Integral/1(x_hat) -> Scope1/1, x_hat/1, Gain/1, Gain5/1
  Sum1/1 -> Switch1/3
  Sum/1 -> Switch1/1
  Gain/1 -> Sum/3
  Gain5/1 -> Sum1/3
  Matrix Multiply/1 -> Sum/2, Sum1/2
  MatrizesA8/1 -> Sum1/1, Sum/1
  Lobs/1 -> Matrix Multiply/1
  rsign/1 -> Matrix Multiply/2

== system boostObserver_old/reset/Augmented Error Generator/z1 ==
  z_dot : Inport
  Constant1 : Constant  Value=[0;0]  VectorParams1D=off
  Gain2 : Gain  Gain=Cmatrix  Multiplication=Matrix(K*u) (u vector)
  Integrator6 : Integrator  InitialConditionSource=external
  z : Outport
  wires:
  Gain2/1 -> Integrator6/1
  Integrator6/1 -> z/1
  z_dot/1 -> Gain2/1
  Constant1/1 -> Integrator6/2

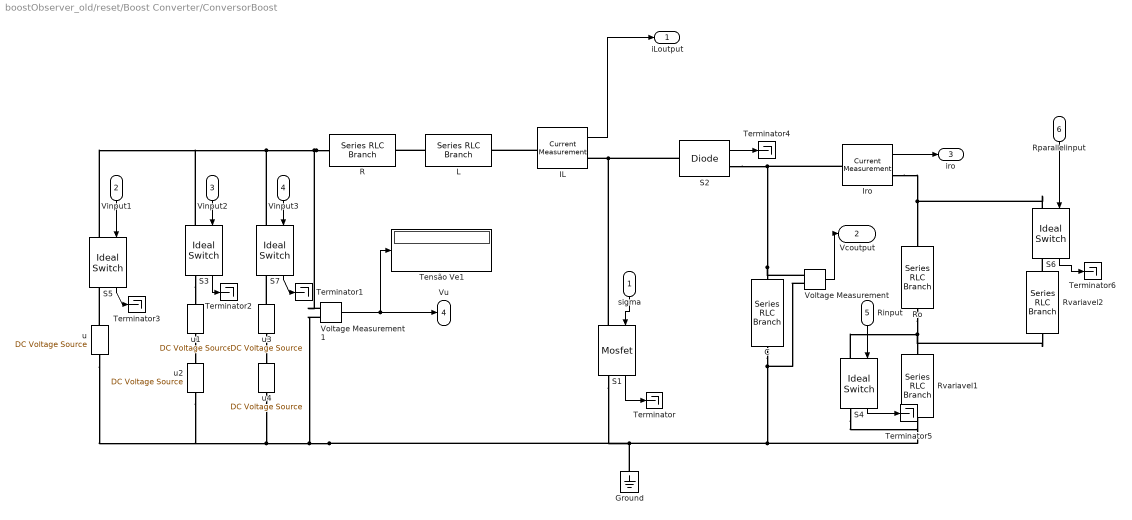
== system boostObserver_old/reset/Boost Converter/ConversorBoost ==
  sigma : Inport
  Vinput1 : Inport  Port=2
  Vinput2 : Inport  Port=3
  Vinput3 : Inport  Port=4
  Rinput : Inport  Port=5
  Rparallelinput : Inport  Port=6
  C : powerlib/Elements/Series RLC Branch  LConnTagsString=__new0  RConnTagsString=__new0  BranchType=C  Resistance=1  Inductance=1e-3  SetiL0=off  InitialCurrent=0  Capacitance=C  Setx0=on  InitialVoltage=0  Measurements=None
  Ground : powerlib/Elements/Ground  LConnTagsString=a
  IL : powerlib/Measurements/Current Measurement  PhasorSimulation=off  OutputType=Complex  PSBequivalent=0
  Iro : powerlib/Measurements/Current Measurement  PhasorSimulation=off  OutputType=Complex  PSBequivalent=0
  L : powerlib/Elements/Series RLC Branch  LConnTagsString=__new0  RConnTagsString=__new0  BranchType=L  Resistance=1  Inductance=L  SetiL0=on  InitialCurrent=0  Capacitance=1e-6  Setx0=off  InitialVoltage=0  Measurements=None
  R : powerlib/Elements/Series RLC Branch  LConnTagsString=__new0  RConnTagsString=__new0  BranchType=R  Resistance=R  Inductance=1e-3  SetiL0=off  InitialCurrent=0  Capacitance=1e-6  Setx0=off  InitialVoltage=0  Measurements=None
  Ro : powerlib/Elements/Series RLC Branch  LConnTagsString=__new0  RConnTagsString=__new0  BranchType=R  Resistance=Ro  Inductance=1e-3  SetiL0=off  InitialCurrent=0  Capacitance=1e-6  Setx0=off  InitialVoltage=0  Measurements=None
  Rvariavel1 : powerlib/Elements/Series RLC Branch  LConnTagsString=__new0  RConnTagsString=__new0  BranchType=R  Resistance=LoadAddResistor  Inductance=1e-3  SetiL0=off  InitialCurrent=0  Capacitance=1e-6  Setx0=off  InitialVoltage=0  Measurements=None
  Rvariavel2 : powerlib/Elements/Series RLC Branch  LConnTagsString=__new0  RConnTagsString=__new0  BranchType=R  Resistance=LoadRemoveResistor  Inductance=1e-3  SetiL0=off  InitialCurrent=0  Capacitance=1e-6  Setx0=off  InitialVoltage=0  Measurements=None
  S1 : powerlib/Power Electronics/Mosfet  Ron=0.0000001  Lon=0  Rd=0.000000001  Vfd=0  IC=0  Rs=1e5  Cs=inf  Measurements=on
  S2 : powerlib/Power Electronics/Diode  Ron=0.000001  Lon=0  Vf=0  IC=0  UseSnubber=off  Rs=0  Cs=0  Measurements=on
  S{3..7} (5 alike) : powerlib/Power Electronics/Ideal Switch  Ron=0.0000001  Lon=0  IC=0  Rs=1e8  Cs=inf  Measurements=on
  Tensão Ve1 : Display
  Terminator{,1..6} (7 alike) : Terminator
  Voltage Measurement : powerlib/Measurements/Voltage Measurement  PhasorSimulation=off  OutputType=Complex  PSBequivalent=0
  Voltage Measurement1 : powerlib/Measurements/Voltage Measurement  PhasorSimulation=off  OutputType=Complex  PSBequivalent=0
  u : powerlib/Electrical Sources/DC Voltage Source  Amplitude=u  Measurements=None
  u1 : powerlib/Electrical Sources/DC Voltage Source  Amplitude=SourceAddVoltage  Measurements=None
  u2 : powerlib/Electrical Sources/DC Voltage Source  Amplitude=u  Measurements=None
  u3 : powerlib/Electrical Sources/DC Voltage Source  Amplitude=SourceRemoveVoltage  Measurements=None
  u4 : powerlib/Electrical Sources/DC Voltage Source  Amplitude=u  Measurements=None
  iLoutput : Outport
  Vcoutput : Outport  Port=2
  iro : Outport  Port=3
  Vu : Outport  Port=4
  wires:
  Rinput/1 -> S4/1
  IL/1 -> iLoutput/1
  sigma/1 -> S1/1
  Voltage Measurement/1 -> Vcoutput/1
  Iro/1 -> iro/1
  Voltage Measurement1/1 -> Vu/1, Tensão Ve1/1
  Vinput1/1 -> S5/1
  Vinput2/1 -> S3/1
  Rparallelinput/1 -> S6/1
  Vinput3/1 -> S7/1
  S1/1 -> Terminator/1
  S7/1 -> Terminator1/1
  S3/1 -> Terminator2/1
  S5/1 -> Terminator3/1
  S2/1 -> Terminator4/1
  S4/1 -> Terminator5/1
  S6/1 -> Terminator6/1
  connections:
  Ro/RConn1 -- Rvariavel2/LConn1 -- Rvariavel1/RConn1 -- S4/LConn1
  IL/LConn1 -- L/RConn1
  C/RConn1 -- S4/RConn1 -- Rvariavel1/LConn1 -- S1/RConn1 -- u2/LConn1 -- u/LConn1 -- u4/LConn1 -- Voltage Measurement1/LConn2 -- Ground/LConn1 -- Voltage Measurement/LConn2
  S2/LConn1 -- S1/LConn1 -- IL/RConn1
  R/LConn1 -- S3/LConn1 -- S5/LConn1 -- S7/LConn1 -- Voltage Measurement1/LConn1
  Iro/RConn1 -- S6/LConn1 -- Ro/LConn1
  L/LConn1 -- R/RConn1
  S2/RConn1 -- Iro/LConn1 -- Voltage Measurement/LConn1 -- C/LConn1
  u/RConn1 -- S5/RConn1
  Rvariavel2/RConn1 -- S6/RConn1
  S3/RConn1 -- u1/RConn1
  u1/LConn1 -- u2/RConn1
  u3/LConn1 -- S7/RConn1
  u3/RConn1 -- u4/RConn1

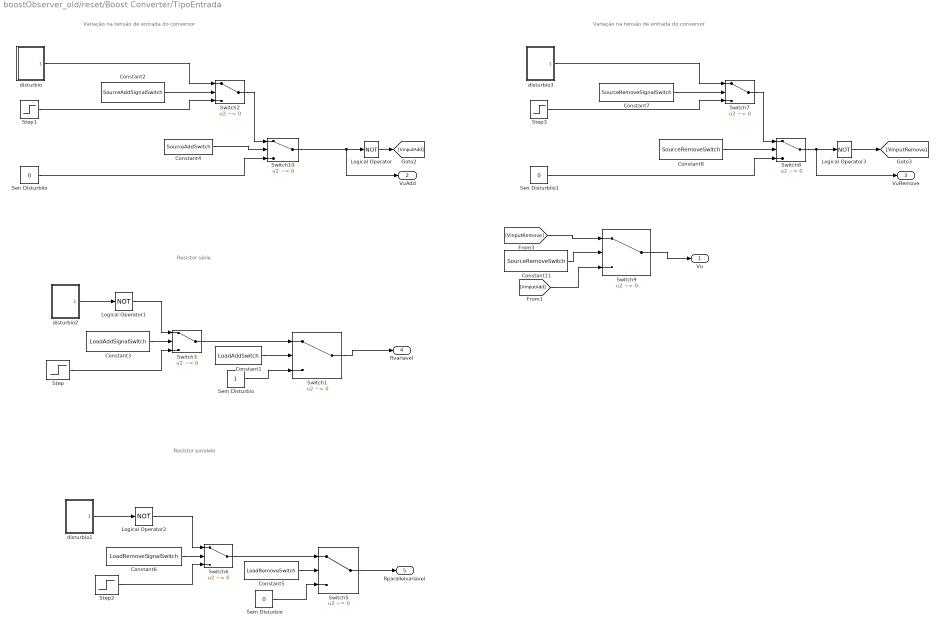
== system boostObserver_old/reset/Boost Converter/TipoEntrada ==
  note: Variação na tensão de entrada do conversor
  note: Resistor série
  note: Resistor paralelo
  note: Variação na tensão de entrada do conversor
  Constant1 : Constant  Value=LoadAddSwitch
  Constant11 : Constant  Value=SourceRemoveSwitch
  Constant2 : Constant  Value=SourceAddSignalSwitch
  Constant3 : Constant  Value=LoadAddSignalSwitch
  Constant4 : Constant  Value=SourceAddSwitch
  Constant5 : Constant  Value=LoadRemoveSwitch
  Constant6 : Constant  Value=LoadRemoveSignalSwitch
  Constant7 : Constant  Value=SourceRemoveSignalSwitch
  Constant8 : Constant  Value=SourceRemoveSwitch
  Logical Operator{,1..3} (4 alike) : Logic  Operator=NOT  AllPortsSameDT=off  OutDataTypeStr=boolean
  Sem Disturbio : Constant
  "Sem Disturbio  " : Constant  Value=0
  Sen Disturbiio : Constant  Value=0
  Sen Disturbiio1 : Constant  Value=0
  Step : Step  Time=LoadAddTime  Before=1  After=0  SampleTime=0
  Step1 : Step  Time=SourceAddTime  SampleTime=0
  Step2 : Step  Time=LoadRemoveTime  SampleTime=0
  Step3 : Step  Time=SourceRemoveTime  SampleTime=0
  Switch{1..3,5..10} (9 alike) : Switch  Criteria=u2 ~= 0
  disturbio : Subsystem
  disturbio1 : Subsystem
  disturbio2 : Subsystem
  disturbio3 : Subsystem
  Vu : Outport
  VuAdd : Outport  Port=2
  VuRemove : Outport  Port=3
  "Rvariavel " : Outport  Port=4
  "Rparallelvariavel " : Outport  Port=5
  wires:
  Sen Disturbiio/1 -> Switch10/3
  Constant4/1 -> Switch10/2
  Constant1/1 -> Switch1/2
  Switch1/1 -> "Rvariavel "/1
  Constant2/1 -> Switch2/2
  Constant3/1 -> Switch3/2
  Switch2/1 -> Switch10/1
  disturbio2/1(disturbio) -> Logical Operator1/1
  Switch3/1 -> Switch1/1
  Sem Disturbio/1 -> Switch1/3
  Switch6/1 -> Switch5/1
  disturbio1/1(disturbio) -> Logical Operator2/1
  Constant6/1 -> Switch6/2
  "Sem Disturbio  "/1 -> Switch5/3
  Switch5/1 -> "Rparallelvariavel "/1
  Constant5/1 -> Switch5/2
  disturbio/1(disturbio) -> Switch2/1
  Step1/1 -> Switch2/3
  Logical Operator1/1 -> Switch3/1
  Step/1 -> Switch3/3
  Step2/1 -> Switch6/3
  Logical Operator2/1 -> Switch6/1
  disturbio3/1(disturbio) -> Switch7/1
  Constant8/1 -> Switch8/2
  Constant7/1 -> Switch7/2
  Switch8/1 -> VuRemove/1, Logical Operator3/1
  Sen Disturbiio1/1 -> Switch8/3
  Switch7/1 -> Switch8/1
  Step3/1 -> Switch7/3
  [VinputAdd] -> Switch9/3
  Constant11/1 -> Switch9/2
  Switch10/1 -> VuAdd/1, Logical Operator/1
  Switch9/1 -> Vu/1
  Logical Operator/1 -> [VinputAdd]
  Logical Operator3/1 -> [VinputRemove]
  [VinputRemove] -> Switch9/1

== system boostObserver_old/reset/Controlador1/SlidingSurface ==
  S : Inport
  ep : Inport  Port=2
  Abs : Abs
  GreaterThan : RelationalOperator  Operator=>  OutDataTypeStr=boolean  RndMeth=Simplest
  If : If  IfExpression=u1 ~= 0
  If Action Subsystem : Subsystem  TreatAsAtomicUnit=on
  If Action Subsystem2 : Subsystem  TreatAsAtomicUnit=on
  Merge1 : Merge
  d : Outport
  wires:
  If Action Subsystem2/1(d) -> Merge1/2
  [S] -> If Action Subsystem/1(S), If Action Subsystem2/1(S)
  If/2 -> If Action Subsystem2/Action
  If/1 -> If Action Subsystem/Action
  [ep] -> If Action Subsystem2/2(ep)
  S/1 -> [S], Abs/1
  If Action Subsystem/1(d) -> Merge1/1
  Abs/1 -> GreaterThan/1
  GreaterThan/1 -> If/1
  Merge1/1 -> d/1
  ep/1 -> [ep], GreaterThan/2
